simulink model "ImuCalibrator3Pass"  (R2018a)
settings: Solver=FixedStepDiscrete  StartTime=0.0  StopTime=inf  FixedStep=1/Fss  RelTol=1e-3
PreLoadFcn:
  | busDef
  | Fss = 1125;
  | Fss = 2100;
InitFcn:
  | modelDef = getModelDef(true);
undefined symbols (not defined in the file or in its folder): df, dw, Ggyr, Macc, Mgyr, numStates
libraries: simulink x15, vrlib x15, dspsigops x6, dspindex x6, dspinverses x6, dspstat3 x3, simulink_extras x3, dspmtrx3 x3, dspsrcs4 x3, dspmathops x3, dspswit3 x1
(part 2 of 4)

== system ImuCalibrator3Pass/firstPass/AINS/gravity meas update ==
  note: this is just to enforce block execution order
  In1 : Inport
  f_ib^b : Inport  Port=2
  stilltime : Inport  Port=3
  Constant : Constant  Value=eye(3)
  Data Store Read1 : DataStoreRead  DataStoreName=Cbn
  Data Store Read3 : DataStoreRead  DataStoreName=P
  Data Store Write : DataStoreWrite  DataStoreName=P
  MATLAB Function1 : MATLAB Function  TreatAsAtomicUnit=on
  MATLAB Function2 : MATLAB Function  TreatAsAtomicUnit=on
  MATLAB Function3 : MATLAB Function  TreatAsAtomicUnit=on
  Math Function : Math  Operator=reciprocal  SaturateOnIntegerOverflow=on
  Math Function1 : Math  Operator=square  SaturateOnIntegerOverflow=on
  Pad : dspsigops/Pad  padAlong=Rows  dimsToPad=1  valSrc=Specify via dialog  padVal=0  spec=Output size  padNumOutRowsSpecMethod=User-specified  numOutRows=1  padNumOutColsSpecMethod=User-specified  numOutCols=numStates  isVarDimsMode=off  padBeginning=0  padEnd=0  outSizeMode=User-specified  outSize=1  padSigAt=End  trunc_flag=None  roundingMode=Floor  overflowMode=off  truncOrWrapMode=Truncate  wrap_flag=None
      settings: SourceProductName=DSP System Toolbox  SourceProductBaseCode=DS
  Permute Dimensions : PermuteDimensions
  Product : Product  Multiplication=Matrix(*)
  Product1 : Product  Multiplication=Matrix(*)
  Product2 : Product
  Product3 : Product  Multiplication=Matrix(*)
  Saturation : Saturate  UpperLimit=9.8*4  LowerLimit=1
  Sum1 : Sum  Inputs=|+-
  "specific force at rest is up, which is -z in NED frame" : Constant  Value=[ 0; 0; -9.8]
  update the Cbn and b_g with the errors : Subsystem
  Out1 : Outport
  wires:
  In1/1 -> Out1/1
  f_ib^b/1 -> Sum1/1  "when still,  z = Cnb*[0 0 -9.8]' + v"
  Data Store Read1/1 -> Permute Dimensions/1  "Cbn hat"
  Permute Dimensions/1 -> Product3/1, Product/1  "Cnb hat"
  Product/1 -> Sum1/2  "zhat"
  Sum1/1 -> Product1/2  "nu = z-zhat"
  MATLAB Function3/1(Pplus) -> Data Store Write/1
  Product3/1 -> Pad/1
  "specific force at rest is up, which is -z in NED frame"/1 -> MATLAB Function2/1(inp_vr), Product/2
  MATLAB Function2/1(res) -> Product3/2
  Data Store Read3/1 -> MATLAB Function3/1(P), MATLAB Function1/1(P)
  Product2/1 -> MATLAB Function3/4(R), MATLAB Function1/3(R)
  Product1/1 -> update the Cbn and b_g with the errors/1(" error state estimates")  "errors"
  Constant/1 -> Product2/1
  Math Function/1 -> Saturation/1
  Saturation/1 -> Math Function1/1
  stilltime/1 -> Math Function/1
  Math Function1/1 -> Product2/2
  Pad/1 -> MATLAB Function3/3(H), MATLAB Function1/2(H)
  MATLAB Function1/2(K) -> Product1/1, MATLAB Function3/2(K)

== system ImuCalibrator3Pass/firstPass/AINS/initialize states and covariances ==
  stilltime : Inport
  f^b : Inport  Port=2
  Compare To Constant : simulink/Logic and Bit Operations/Compare To Constant  relop=>  const=1.0  OutDataTypeStr=boolean
  Data Store Memory : DataStoreMemory  DataStoreName=INITIALIZED  ReadBeforeWriteMsg=warning  WriteAfterWriteMsg=warning  WriteAfterReadMsg=warning  ShowAdditionalParam=off
  Data Store Read : DataStoreRead  DataStoreName=INITIALIZED
  INITIALIZED = 1 : Subsystem
  Logical Operator : Logic  AllPortsSameDT=off  OutDataTypeStr=boolean
  Logical Operator1 : Logic  Operator=NOT  Inputs=1  IconShape=distinctive  AllPortsSameDT=off  OutDataTypeStr=boolean
  calc Cbn : Subsystem  TreatAsAtomicUnit=on
  set P : Subsystem
  set states : Subsystem  TreatAsAtomicUnit=on
  initializing : Outport
  wires:
  Compare To Constant/1 -> Logical Operator/2
  stilltime/1 -> Compare To Constant/1
  Data Store Read/1 -> Logical Operator1/1
  Logical Operator1/1 -> Logical Operator/1
  f^b/1 -> calc Cbn/1(f^b)
  calc Cbn/2(Cbn) -> set states/1(Cbn)
  INITIALIZED = 1/1(Out1) -> initializing/1
  Logical Operator/1 -> calc Cbn/Enable
  calc Cbn/1(Out1) -> set states/Enable
  set states/1(Out1) -> set P/Enable
  set P/1(Out1) -> INITIALIZED = 1/Enable

== system ImuCalibrator3Pass/firstPass/AINS/report output ==
  In1 : Inport
  w_comp : Inport  Port=2
  f_comp : Inport  Port=3
  Dt : Inport  Port=4
  stilltime : Inport  Port=5
  Bus Creator : BusCreator  Inputs=14
  Data Store Read : DataStoreRead  DataStoreName=Cbn
  Data Store Read1 : DataStoreRead  DataStoreName=P
  Data Store Read2 : DataStoreRead  DataStoreName=dw
  Data Store Read3 : DataStoreRead  DataStoreName=rnav
  Data Store Read4 : DataStoreRead  DataStoreName=vnav
  Data Store Read5 : DataStoreRead  DataStoreName=df
  Data Store Read6 : DataStoreRead  DataStoreName=Mgyr
  Data Store Read7 : DataStoreRead  DataStoreName=Macc
  Data Store Read8 : DataStoreRead  DataStoreName=Ggyr
  Extract Diagonal : dspmtrx3/Extract Diagonal
      settings: SourceProductName=DSP System Toolbox  SourceProductBaseCode=DS
  MATLAB Function1 : MATLAB Function  TreatAsAtomicUnit=on
  MATLAB Function3 : MATLAB Function  TreatAsAtomicUnit=on
  Reshape : Reshape  OutputDimensionality=Column vector (2-D)
  Sqrt : Sqrt  SaturateOnIntegerOverflow=on
  Terminator : Terminator
  filterOut : Outport
  wires:
  Data Store Read/1 -> MATLAB Function1/1(Cbn), MATLAB Function3/1(Cbn)
  Extract Diagonal/1 -> Sqrt/1
  Data Store Read1/1 -> Extract Diagonal/1
  In1/1 -> Terminator/1
  Bus Creator/1 -> filterOut/1
  Data Store Read6/1 -> Bus Creator/10  "Mgyr"
  Sqrt/1 -> Reshape/1  "sigmas"
  f_comp/1 -> Bus Creator/9  "f_comp"
  Data Store Read8/1 -> Bus Creator/12  "Ggyr"
  Data Store Read5/1 -> Bus Creator/6  "df"
  w_comp/1 -> Bus Creator/8  "w_comp"
  Data Store Read4/1 -> Bus Creator/5  "vnav"
  Data Store Read2/1 -> Bus Creator/3  "dw"
  Data Store Read3/1 -> Bus Creator/4  "rnav"
  MATLAB Function3/1(eul) -> Bus Creator/2  "eulers"
  Data Store Read7/1 -> Bus Creator/11  "Macc"
  MATLAB Function1/1(quat) -> Bus Creator/1  "quaternion"
  Dt/1 -> Bus Creator/13  "Dt"
  stilltime/1 -> Bus Creator/14  "stilltime"
  Reshape/1 -> Bus Creator/7  "sigmas"

== system ImuCalibrator3Pass/firstPass/AINS/sensor compensation ==
  note: w_meas = w_true + dw + Mgyr * w_true + Ggyr * f_true
      | w_comp = (I + Mgyr) -1 * (w_meas - dw - Ggyr * f_true)
      |
      | f_meas = f_true + df + Macc * f_true
      | f_comp = (I + Macc) -1 * (f_meas - df)
  w_ib^b : Inport  Unit=rad/s
  f_ib^b : Inport  Port=2  Unit=m/s^2  PortDimensions=3
  Dt : Inport  Port=3  Unit=rad/s
  Data Store Read : DataStoreRead  DataStoreName=IplusMinv_gyr
  Data Store Read1 : DataStoreRead  DataStoreName=dw
  Data Store Read2 : DataStoreRead  DataStoreName=IplusMinv_acc
  Data Store Read3 : DataStoreRead  DataStoreName=df
  Data Store Read4 : DataStoreRead  DataStoreName=Ggyr
  Product : Product  Multiplication=Matrix(*)
  Product1 : Product  Multiplication=Matrix(*)
  Product2 : Product  Multiplication=Matrix(*)
  Sum : Sum  Inputs=|+-
  Sum1 : Sum  Inputs=|+-
  Sum2 : Sum  Inputs=|+-
  w_comp : Outport
  f_comp : Outport  Port=2
  DtOut : Outport  Port=3
  wires:
  Dt/1 -> DtOut/1
  Data Store Read1/1 -> Sum/2
  w_ib^b/1 -> Sum/1
  Sum/1 -> Sum2/1
  Data Store Read/1 -> Product/1
  Product/1 -> w_comp/1
  Product1/1 -> Product2/2, f_comp/1
  Data Store Read2/1 -> Product1/1
  Sum1/1 -> Product1/2
  f_ib^b/1 -> Sum1/1
  Data Store Read3/1 -> Sum1/2
  Sum2/1 -> Product/2
  Product2/1 -> Sum2/2
  Data Store Read4/1 -> Product2/1

== system ImuCalibrator3Pass/firstPass/AINS/time update ==
  Cbn : Inport
  Dt : Inport  Port=2
  w : Inport  Port=3
  f : Inport  Port=4
  Constant : Constant  Commented=on  Value=numStates
  Data Store Read : DataStoreRead  DataStoreName=P
  Data Store Read1 : DataStoreRead  DataStoreName=Cbn
  Data Store Write : DataStoreWrite  DataStoreName=P
  MATLAB Function : MATLAB Function  TreatAsAtomicUnit=on
  MATLAB Function1 : MATLAB Function  Commented=on  TreatAsAtomicUnit=on
  MATLAB Function2 : MATLAB Function  Commented=on  TreatAsAtomicUnit=on
  MATLAB Function3 : MATLAB Function  TreatAsAtomicUnit=on
  Permute Dimensions : PermuteDimensions
  Product2 : Product  Inputs=3  Multiplication=Matrix(*)
  Sum : Sum  Inputs=|++
  Out1 : Outport
  wires:
  Cbn/1 -> Out1/1  "this is just to enforce block execution order"
  Dt/1 -> MATLAB Function3/3(Dt), MATLAB Function/3(Dt)
  MATLAB Function3/1(Phi) -> Permute Dimensions/1, Product2/1  "Phi"
  Data Store Read/1 -> Product2/2
  Permute Dimensions/1 -> Product2/3  "Phi'"
  Sum/1 -> Data Store Write/1  "Phi*P*Phi' + Q"
  Data Store Read1/1 -> MATLAB Function3/4(Cbn), MATLAB Function/4(Cbn)
  w/1 -> MATLAB Function3/1(omega), MATLAB Function/1(omega)
  f/1 -> MATLAB Function3/2(fbod), MATLAB Function/2(f_ib)
  Constant/1 -> MATLAB Function2/1(numStates)
  MATLAB Function/1(Q) -> Sum/2
  Product2/1 -> Sum/1  "Phi*P*Phi'"

== system ImuCalibrator3Pass/firstPass/AINS/zero velocity update ==
  note: this is just to enforce block execution order
  In1 : Inport
  stilltime : Inport  Port=2
  0.01s to 10s : Saturate  UpperLimit=10  LowerLimit=0.01
  Constant : Constant  Value=eye(3)
  Constant1 : Constant  Value=eye(3)
  Constant2 : Constant  Value=zeros(3,9)  VectorParams1D=off
  Constant3 : Constant  Value=zeros(3,1)  VectorParams1D=off
  Data Store Read1 : DataStoreRead  DataStoreName=vnav
  Data Store Read3 : DataStoreRead  DataStoreName=P
  Data Store Write : DataStoreWrite  DataStoreName=P
  MATLAB Function1 : MATLAB Function  TreatAsAtomicUnit=on
  MATLAB Function3 : MATLAB Function  TreatAsAtomicUnit=on
  Math Function : Math  Operator=reciprocal  SaturateOnIntegerOverflow=on
  Math Function1 : Math  Operator=square  SaturateOnIntegerOverflow=on
  Matrix Concatenate : Concatenate  Mode=Multidimensional array  ConcatenateDimension=2
  Pad : dspsigops/Pad  padAlong=Rows  dimsToPad=1  valSrc=Specify via dialog  padVal=0  spec=Output size  padNumOutRowsSpecMethod=User-specified  numOutRows=1  padNumOutColsSpecMethod=User-specified  numOutCols=modelDef.numStates  isVarDimsMode=off  padBeginning=0  padEnd=0  outSizeMode=User-specified  outSize=1  padSigAt=End  trunc_flag=None  roundingMode=Floor  overflowMode=off  truncOrWrapMode=Truncate  wrap_flag=None
      settings: SourceProductName=DSP System Toolbox  SourceProductBaseCode=DS
  Product1 : Product  Multiplication=Matrix(*)
  Product2 : Product
  Saturation : Saturate  UpperLimit=100  LowerLimit=0.1
  Scope : Scope
  Scope1 : Scope
  Sum1 : Sum  Inputs=|+-
  update the underlying states : Subsystem
  Out1 : Outport
  wires:
  MATLAB Function1/2(K) -> Product1/1, MATLAB Function3/2(K)
  Pad/1 -> MATLAB Function1/2(H), MATLAB Function3/3(H)
  Math Function1/1 -> Product2/2
  stilltime/1 -> 0.01s to 10s/1
  Saturation/1 -> Scope/1, Math Function1/1
  Math Function/1 -> Saturation/1
  Constant/1 -> Product2/1
  Product1/1 -> update the underlying states/1(" error state estimates")  "errors"
  Product2/1 -> MATLAB Function1/3(R), MATLAB Function3/4(R)
  Data Store Read3/1 -> MATLAB Function1/1(P), MATLAB Function3/1(P)
  Matrix Concatenate/1 -> Pad/1
  MATLAB Function3/1(Pplus) -> Data Store Write/1
  Sum1/1 -> Scope1/1, Product1/2  "nu = dv = vhat - vtrue"
  In1/1 -> Out1/1
  Constant2/1 -> Matrix Concatenate/1
  Constant1/1 -> Matrix Concatenate/2
  0.01s to 10s/1 -> Math Function/1
  Data Store Read1/1 -> Sum1/1
  Constant3/1 -> Sum1/2

== system ImuCalibrator3Pass/firstPass/readImuData/write SensorTypeIdentifier once ==
  In1 : Inport
  Enable : EnablePort
  Data Store Write : DataStoreWrite  DataStoreName=SensorTypeIdentifier
  wires:
  In1/1 -> Data Store Write/1

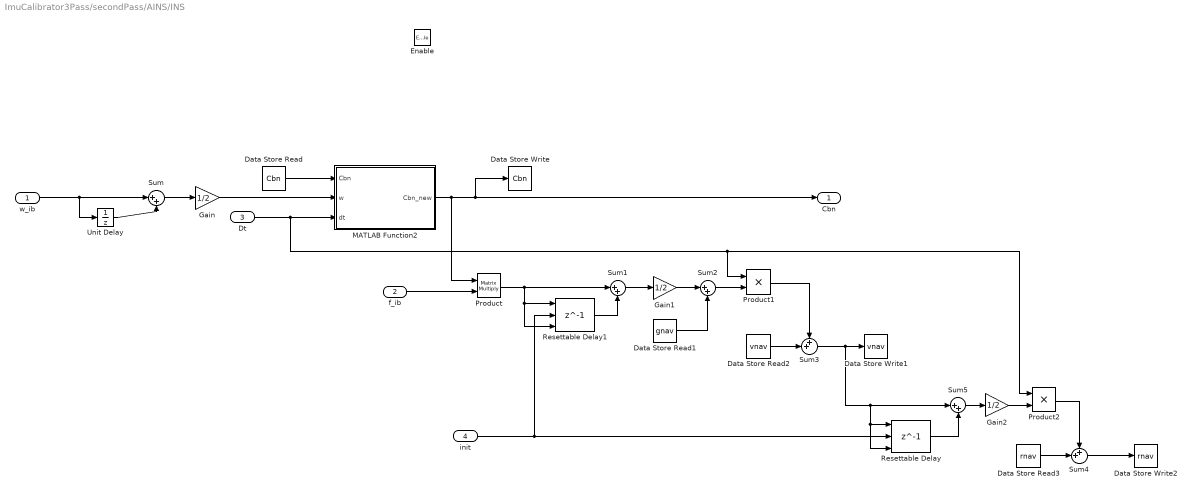
== system ImuCalibrator3Pass/secondPass/AINS/INS ==
  w_ib : Inport
  f_ib : Inport  Port=2
  Dt : Inport  Port=3
  init : Inport  Port=4
  Enable : EnablePort
  Data Store Read : DataStoreRead  DataStoreName=Cbn
  Data Store Read1 : DataStoreRead  DataStoreName=gnav
  Data Store Read2 : DataStoreRead  DataStoreName=vnav
  Data Store Read3 : DataStoreRead  DataStoreName=rnav
  Data Store Write : DataStoreWrite  DataStoreName=Cbn
  Data Store Write1 : DataStoreWrite  DataStoreName=vnav
  Data Store Write2 : DataStoreWrite  DataStoreName=rnav
  Gain : Gain  Gain=1/2
  Gain1 : Gain  Gain=1/2
  Gain2 : Gain  Gain=1/2
  MATLAB Function2 : MATLAB Function  TreatAsAtomicUnit=on
  Product : Product  Multiplication=Matrix(*)
  Product1 : Product
  Product2 : Product
  Resettable Delay : Delay  DelayLength=1  InitialConditionSource=Input port  ExternalReset=Level
      settings: InputPortMap=u0,r5,p4
  Resettable Delay1 : Delay  DelayLength=1  InitialConditionSource=Input port  ExternalReset=Level
      settings: InputPortMap=u0,r5,p4
  Sum{,1..2,5} (4 alike) : Sum  Inputs=|++
  Sum3 : Sum  Inputs=++|
  Sum4 : Sum  Inputs=++|
  Unit Delay : UnitDelay  SampleTime=-1
  Cbn : Outport
  wires:
  Product2/1 -> Sum4/1
  Resettable Delay1/1 -> Sum1/2
  init/1 -> Resettable Delay/2, Resettable Delay1/2
  Resettable Delay/1 -> Sum5/2
  Gain2/1 -> Product2/2
  Sum3/1 -> Data Store Write1/1, Sum5/1, Resettable Delay/1, Resettable Delay/3
  Sum5/1 -> Gain2/1
  Sum4/1 -> Data Store Write2/1
  Data Store Read3/1 -> Sum4/2
  Product1/1 -> Sum3/1
  Data Store Read2/1 -> Sum3/2
  Gain1/1 -> Sum2/1
  Sum1/1 -> Gain1/1
  Product/1 -> Sum1/1, Resettable Delay1/1, Resettable Delay1/3
  Sum2/1 -> Product1/2
  Data Store Read1/1 -> Sum2/2
  f_ib/1 -> Product/2
  Gain/1 -> MATLAB Function2/2(w)
  Sum/1 -> Gain/1
  Unit Delay/1 -> Sum/2
  MATLAB Function2/1(Cbn_new) -> Data Store Write/1, Cbn/1, Product/1
  w_ib/1 -> Sum/1, Unit Delay/1
  Data Store Read/1 -> MATLAB Function2/1(Cbn)
  Dt/1 -> MATLAB Function2/3(dt), Product1/1, Product2/1

== system ImuCalibrator3Pass/secondPass/AINS/compass meas update ==
  note: this is just to enforce block execution order
  In1 : Inport
  m^b : Inport  Port=2
  Enable : EnablePort
  Data Store Read1 : DataStoreRead  DataStoreName=Cbn
  Data Store Read3 : DataStoreRead  DataStoreName=P
  Data Store Write : DataStoreWrite  DataStoreName=P
  Demux : Demux  Outputs=3
  Gain : Gain  Gain=-1
  H : Constant  Value=[ 0 0 1]  VectorParams1D=off
  MATLAB Function1 : MATLAB Function  TreatAsAtomicUnit=on
  MATLAB Function3 : MATLAB Function  TreatAsAtomicUnit=on
  Product : Product  Multiplication=Matrix(*)
  Product1 : Product  Multiplication=Matrix(*)
  R assumes 10 deg rms compass noise : Constant  Value=0.34^2
  Scope : Scope
  Scope1 : Scope
  Scope2 : Scope
  Trigonometric Function : Trigonometry  Operator=atan2
  update the Cbn with the errors : Subsystem
  Out1 : Outport
  wires:
  Gain/1 -> Scope1/1, Product1/2
  H/1 -> MATLAB Function3/3(H), MATLAB Function1/2(H)
  Demux/1 -> Trigonometric Function/2
  Demux/2 -> Trigonometric Function/1
  In1/1 -> Out1/1
  Data Store Read1/1 -> Product/1  "Cbn hat"
  Product/1 -> Demux/1  "m^nhat"
  Trigonometric Function/1 -> Gain/1  "nu = 0 - psi"
  MATLAB Function1/2(K) -> Scope2/1, MATLAB Function3/2(K), Product1/1
  MATLAB Function3/1(Pplus) -> Data Store Write/1
  m^b/1 -> Product/2
  Data Store Read3/1 -> MATLAB Function3/1(P), MATLAB Function1/1(P)
  R assumes 10 deg rms compass noise/1 -> MATLAB Function3/4(R), MATLAB Function1/3(R)
  Product1/1 -> Scope/1, update the Cbn with the errors/1(phi  rotation errors)  "phi  rotation errors"

== system ImuCalibrator3Pass/secondPass/AINS/gravity meas update ==
  note: this is just to enforce block execution order
  In1 : Inport
  f_ib^b : Inport  Port=2
  stilltime : Inport  Port=3
  Constant : Constant  Value=eye(3)
  Data Store Read1 : DataStoreRead  DataStoreName=Cbn
  Data Store Read3 : DataStoreRead  DataStoreName=P
  Data Store Write : DataStoreWrite  DataStoreName=P
  MATLAB Function1 : MATLAB Function  TreatAsAtomicUnit=on
  MATLAB Function2 : MATLAB Function  TreatAsAtomicUnit=on
  MATLAB Function3 : MATLAB Function  TreatAsAtomicUnit=on
  Math Function : Math  Operator=reciprocal  SaturateOnIntegerOverflow=on
  Math Function1 : Math  Operator=square  SaturateOnIntegerOverflow=on
  Pad : dspsigops/Pad  padAlong=Rows  dimsToPad=1  valSrc=Specify via dialog  padVal=0  spec=Output size  padNumOutRowsSpecMethod=User-specified  numOutRows=1  padNumOutColsSpecMethod=User-specified  numOutCols=numStates  isVarDimsMode=off  padBeginning=0  padEnd=0  outSizeMode=User-specified  outSize=1  padSigAt=End  trunc_flag=None  roundingMode=Floor  overflowMode=off  truncOrWrapMode=Truncate  wrap_flag=None
      settings: SourceProductName=DSP System Toolbox  SourceProductBaseCode=DS
  Permute Dimensions : PermuteDimensions
  Product : Product  Multiplication=Matrix(*)
  Product1 : Product  Multiplication=Matrix(*)
  Product2 : Product
  Product3 : Product  Multiplication=Matrix(*)
  Saturation : Saturate  UpperLimit=9.8*4  LowerLimit=1
  Sum1 : Sum  Inputs=|+-
  "specific force at rest is up, which is -z in NED frame" : Constant  Value=[ 0; 0; -9.8]
  update the Cbn and b_g with the errors : Subsystem
  Out1 : Outport
  wires:
  MATLAB Function1/2(K) -> MATLAB Function3/2(K), Product1/1
  Pad/1 -> MATLAB Function1/2(H), MATLAB Function3/3(H)
  Math Function1/1 -> Product2/2
  stilltime/1 -> Math Function/1
  Saturation/1 -> Math Function1/1
  Math Function/1 -> Saturation/1
  Constant/1 -> Product2/1
  Product1/1 -> update the Cbn and b_g with the errors/1(" error state estimates")  "errors"
  Product2/1 -> MATLAB Function1/3(R), MATLAB Function3/4(R)
  Data Store Read3/1 -> MATLAB Function1/1(P), MATLAB Function3/1(P)
  MATLAB Function2/1(res) -> Product3/2
  "specific force at rest is up, which is -z in NED frame"/1 -> Product/2, MATLAB Function2/1(inp_vr)
  Product3/1 -> Pad/1
  MATLAB Function3/1(Pplus) -> Data Store Write/1
  Sum1/1 -> Product1/2  "nu = z-zhat"
  Product/1 -> Sum1/2  "zhat"
  Permute Dimensions/1 -> Product/1, Product3/1  "Cnb hat"
  Data Store Read1/1 -> Permute Dimensions/1  "Cbn hat"
  f_ib^b/1 -> Sum1/1  "when still,  z = Cnb*[0 0 -9.8]' + v"
  In1/1 -> Out1/1

== system ImuCalibrator3Pass/secondPass/AINS/initialize states and covariances ==
  stilltime : Inport
  f^b : Inport  Port=2
  Compare To Constant : simulink/Logic and Bit Operations/Compare To Constant  relop=>  const=1.0  OutDataTypeStr=boolean
  Data Store Memory : DataStoreMemory  DataStoreName=INITIALIZED  ReadBeforeWriteMsg=warning  WriteAfterWriteMsg=warning  WriteAfterReadMsg=warning  ShowAdditionalParam=off
  Data Store Read : DataStoreRead  DataStoreName=INITIALIZED
  INITIALIZED = 1 : Subsystem
  Logical Operator : Logic  AllPortsSameDT=off  OutDataTypeStr=boolean
  Logical Operator1 : Logic  Operator=NOT  Inputs=1  IconShape=distinctive  AllPortsSameDT=off  OutDataTypeStr=boolean
  calc Cbn : Subsystem  TreatAsAtomicUnit=on
  set P : Subsystem
  set states : Subsystem  TreatAsAtomicUnit=on
  initializing : Outport
  wires:
  set P/1(Out1) -> INITIALIZED = 1/Enable
  set states/1(Out1) -> set P/Enable
  calc Cbn/1(Out1) -> set states/Enable
  Logical Operator/1 -> calc Cbn/Enable
  INITIALIZED = 1/1(Out1) -> initializing/1
  calc Cbn/2(Cbn) -> set states/1(Cbn)
  f^b/1 -> calc Cbn/1(f^b)
  Logical Operator1/1 -> Logical Operator/1
  Data Store Read/1 -> Logical Operator1/1
  stilltime/1 -> Compare To Constant/1
  Compare To Constant/1 -> Logical Operator/2

== system ImuCalibrator3Pass/secondPass/AINS/report output ==
  In1 : Inport
  w_comp : Inport  Port=2
  f_comp : Inport  Port=3
  Dt : Inport  Port=4
  stilltime : Inport  Port=5
  Bus Creator : BusCreator  Inputs=14
  Data Store Read : DataStoreRead  DataStoreName=Cbn
  Data Store Read1 : DataStoreRead  DataStoreName=P
  Data Store Read2 : DataStoreRead  DataStoreName=dw
  Data Store Read3 : DataStoreRead  DataStoreName=rnav
  Data Store Read4 : DataStoreRead  DataStoreName=vnav
  Data Store Read5 : DataStoreRead  DataStoreName=df
  Data Store Read6 : DataStoreRead  DataStoreName=Mgyr
  Data Store Read7 : DataStoreRead  DataStoreName=Macc
  Data Store Read8 : DataStoreRead  DataStoreName=Ggyr
  Extract Diagonal : dspmtrx3/Extract Diagonal
      settings: SourceProductName=DSP System Toolbox  SourceProductBaseCode=DS
  MATLAB Function1 : MATLAB Function  TreatAsAtomicUnit=on
  MATLAB Function3 : MATLAB Function  TreatAsAtomicUnit=on
  Reshape : Reshape  OutputDimensionality=Column vector (2-D)
  Sqrt : Sqrt  SaturateOnIntegerOverflow=on
  Terminator : Terminator
  filterOut : Outport
  wires:
  Reshape/1 -> Bus Creator/7  "sigmas"
  stilltime/1 -> Bus Creator/14  "stilltime"
  Dt/1 -> Bus Creator/13  "Dt"
  MATLAB Function1/1(quat) -> Bus Creator/1  "quaternion"
  Data Store Read7/1 -> Bus Creator/11  "Macc"
  MATLAB Function3/1(eul) -> Bus Creator/2  "eulers"
  Data Store Read3/1 -> Bus Creator/4  "rnav"
  Data Store Read2/1 -> Bus Creator/3  "dw"
  Data Store Read4/1 -> Bus Creator/5  "vnav"
  w_comp/1 -> Bus Creator/8  "w_comp"
  Data Store Read5/1 -> Bus Creator/6  "df"
  Data Store Read8/1 -> Bus Creator/12  "Ggyr"
  f_comp/1 -> Bus Creator/9  "f_comp"
  Sqrt/1 -> Reshape/1  "sigmas"
  Data Store Read6/1 -> Bus Creator/10  "Mgyr"
  Bus Creator/1 -> filterOut/1
  In1/1 -> Terminator/1
  Data Store Read1/1 -> Extract Diagonal/1
  Extract Diagonal/1 -> Sqrt/1
  Data Store Read/1 -> MATLAB Function3/1(Cbn), MATLAB Function1/1(Cbn)

== system ImuCalibrator3Pass/secondPass/AINS/sensor compensation ==
  note: w_meas = w_true + dw + Mgyr * w_true + Ggyr * f_true
      | w_comp = (I + Mgyr) -1 * (w_meas - dw - Ggyr * f_true)
      |
      | f_meas = f_true + df + Macc * f_true
      | f_comp = (I + Macc) -1 * (f_meas - df)
  w_ib^b : Inport  Unit=rad/s
  f_ib^b : Inport  Port=2  Unit=m/s^2  PortDimensions=3
  Dt : Inport  Port=3  Unit=rad/s
  Data Store Read : DataStoreRead  DataStoreName=IplusMinv_gyr
  Data Store Read1 : DataStoreRead  DataStoreName=dw
  Data Store Read2 : DataStoreRead  DataStoreName=IplusMinv_acc
  Data Store Read3 : DataStoreRead  DataStoreName=df
  Data Store Read4 : DataStoreRead  DataStoreName=Ggyr
  Product : Product  Multiplication=Matrix(*)
  Product1 : Product  Multiplication=Matrix(*)
  Product2 : Product  Multiplication=Matrix(*)
  Sum : Sum  Inputs=|+-
  Sum1 : Sum  Inputs=|+-
  Sum2 : Sum  Inputs=|+-
  w_comp : Outport
  f_comp : Outport  Port=2
  DtOut : Outport  Port=3
  wires:
  Data Store Read4/1 -> Product2/1
  Product2/1 -> Sum2/2
  Sum2/1 -> Product/2
  Data Store Read3/1 -> Sum1/2
  f_ib^b/1 -> Sum1/1
  Sum1/1 -> Product1/2
  Data Store Read2/1 -> Product1/1
  Product1/1 -> f_comp/1, Product2/2
  Product/1 -> w_comp/1
  Data Store Read/1 -> Product/1
  Sum/1 -> Sum2/1
  w_ib^b/1 -> Sum/1
  Data Store Read1/1 -> Sum/2
  Dt/1 -> DtOut/1

== system ImuCalibrator3Pass/secondPass/AINS/time update ==
  Cbn : Inport
  Dt : Inport  Port=2
  w : Inport  Port=3
  f : Inport  Port=4
  Constant : Constant  Commented=on  Value=numStates
  Data Store Read : DataStoreRead  DataStoreName=P
  Data Store Read1 : DataStoreRead  DataStoreName=Cbn
  Data Store Write : DataStoreWrite  DataStoreName=P
  MATLAB Function : MATLAB Function  TreatAsAtomicUnit=on
  MATLAB Function1 : MATLAB Function  Commented=on  TreatAsAtomicUnit=on
  MATLAB Function2 : MATLAB Function  Commented=on  TreatAsAtomicUnit=on
  MATLAB Function3 : MATLAB Function  TreatAsAtomicUnit=on
  Permute Dimensions : PermuteDimensions
  Product2 : Product  Inputs=3  Multiplication=Matrix(*)
  Sum : Sum  Inputs=|++
  Out1 : Outport
  wires:
  Product2/1 -> Sum/1  "Phi*P*Phi'"
  MATLAB Function/1(Q) -> Sum/2
  Constant/1 -> MATLAB Function2/1(numStates)
  f/1 -> MATLAB Function/2(f_ib), MATLAB Function3/2(fbod)
  w/1 -> MATLAB Function/1(omega), MATLAB Function3/1(omega)
  Data Store Read1/1 -> MATLAB Function/4(Cbn), MATLAB Function3/4(Cbn)
  Sum/1 -> Data Store Write/1  "Phi*P*Phi' + Q"
  Permute Dimensions/1 -> Product2/3  "Phi'"
  Data Store Read/1 -> Product2/2
  MATLAB Function3/1(Phi) -> Product2/1, Permute Dimensions/1  "Phi"
  Dt/1 -> MATLAB Function/3(Dt), MATLAB Function3/3(Dt)
  Cbn/1 -> Out1/1  "this is just to enforce block execution order"

== system ImuCalibrator3Pass/secondPass/AINS/zero velocity update ==
  note: this is just to enforce block execution order
  In1 : Inport
  stilltime : Inport  Port=2
  0.01s to 10s : Saturate  UpperLimit=10  LowerLimit=0.01
  Constant : Constant  Value=eye(3)
  Constant1 : Constant  Value=eye(3)
  Constant2 : Constant  Value=zeros(3,9)  VectorParams1D=off
  Constant3 : Constant  Value=zeros(3,1)  VectorParams1D=off
  Data Store Read1 : DataStoreRead  DataStoreName=vnav
  Data Store Read3 : DataStoreRead  DataStoreName=P
  Data Store Write : DataStoreWrite  DataStoreName=P
  MATLAB Function1 : MATLAB Function  TreatAsAtomicUnit=on
  MATLAB Function3 : MATLAB Function  TreatAsAtomicUnit=on
  Math Function : Math  Operator=reciprocal  SaturateOnIntegerOverflow=on
  Math Function1 : Math  Operator=square  SaturateOnIntegerOverflow=on
  Matrix Concatenate : Concatenate  Mode=Multidimensional array  ConcatenateDimension=2
  Pad : dspsigops/Pad  padAlong=Rows  dimsToPad=1  valSrc=Specify via dialog  padVal=0  spec=Output size  padNumOutRowsSpecMethod=User-specified  numOutRows=1  padNumOutColsSpecMethod=User-specified  numOutCols=modelDef.numStates  isVarDimsMode=off  padBeginning=0  padEnd=0  outSizeMode=User-specified  outSize=1  padSigAt=End  trunc_flag=None  roundingMode=Floor  overflowMode=off  truncOrWrapMode=Truncate  wrap_flag=None
      settings: SourceProductName=DSP System Toolbox  SourceProductBaseCode=DS
  Product1 : Product  Multiplication=Matrix(*)
  Product2 : Product
  Saturation : Saturate  UpperLimit=100  LowerLimit=0.1
  Scope : Scope
  Scope1 : Scope
  Sum1 : Sum  Inputs=|+-
  update the underlying states : Subsystem
  Out1 : Outport
  wires:
  Constant3/1 -> Sum1/2
  Data Store Read1/1 -> Sum1/1
  0.01s to 10s/1 -> Math Function/1
  Constant1/1 -> Matrix Concatenate/2
  Constant2/1 -> Matrix Concatenate/1
  In1/1 -> Out1/1
  Sum1/1 -> Product1/2, Scope1/1  "nu = dv = vhat - vtrue"
  MATLAB Function3/1(Pplus) -> Data Store Write/1
  Matrix Concatenate/1 -> Pad/1
  Data Store Read3/1 -> MATLAB Function3/1(P), MATLAB Function1/1(P)
  Product2/1 -> MATLAB Function3/4(R), MATLAB Function1/3(R)
  Product1/1 -> update the underlying states/1(" error state estimates")  "errors"
  Constant/1 -> Product2/1
  Math Function/1 -> Saturation/1
  Saturation/1 -> Math Function1/1, Scope/1
  stilltime/1 -> 0.01s to 10s/1
  Math Function1/1 -> Product2/2
  Pad/1 -> MATLAB Function3/3(H), MATLAB Function1/2(H)
  MATLAB Function1/2(K) -> MATLAB Function3/2(K), Product1/1

== system ImuCalibrator3Pass/secondPass/readImuData/write SensorTypeIdentifier once ==
  In1 : Inport
  Enable : EnablePort
  Data Store Write : DataStoreWrite  DataStoreName=SensorTypeIdentifier
  wires:
  In1/1 -> Data Store Write/1

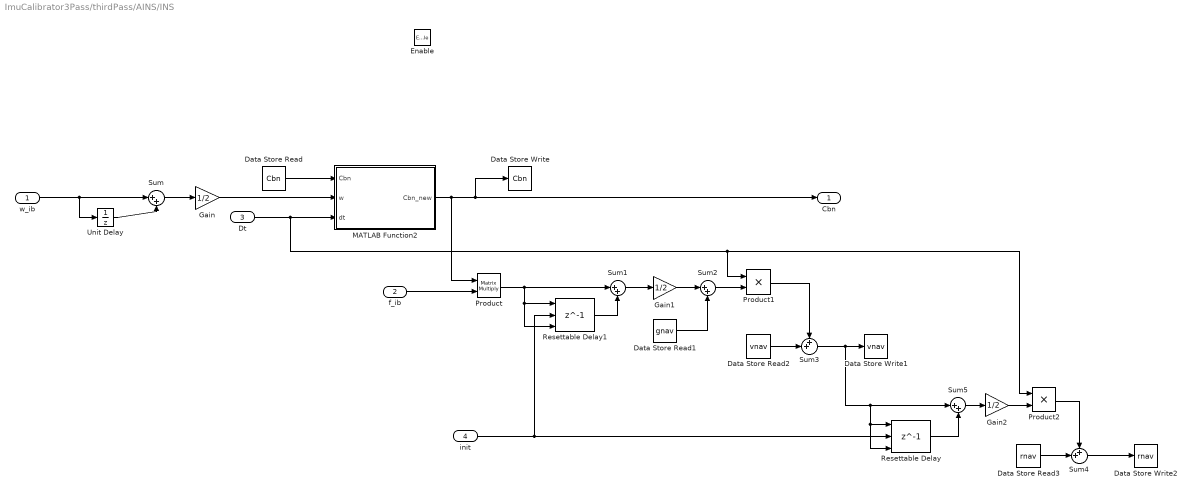
== system ImuCalibrator3Pass/thirdPass/AINS/INS ==
  w_ib : Inport
  f_ib : Inport  Port=2
  Dt : Inport  Port=3
  init : Inport  Port=4
  Enable : EnablePort
  Data Store Read : DataStoreRead  DataStoreName=Cbn
  Data Store Read1 : DataStoreRead  DataStoreName=gnav
  Data Store Read2 : DataStoreRead  DataStoreName=vnav
  Data Store Read3 : DataStoreRead  DataStoreName=rnav
  Data Store Write : DataStoreWrite  DataStoreName=Cbn
  Data Store Write1 : DataStoreWrite  DataStoreName=vnav
  Data Store Write2 : DataStoreWrite  DataStoreName=rnav
  Gain : Gain  Gain=1/2
  Gain1 : Gain  Gain=1/2
  Gain2 : Gain  Gain=1/2
  MATLAB Function2 : MATLAB Function  TreatAsAtomicUnit=on
  Product : Product  Multiplication=Matrix(*)
  Product1 : Product
  Product2 : Product
  Resettable Delay : Delay  DelayLength=1  InitialConditionSource=Input port  ExternalReset=Level
      settings: InputPortMap=u0,r5,p4
  Resettable Delay1 : Delay  DelayLength=1  InitialConditionSource=Input port  ExternalReset=Level
      settings: InputPortMap=u0,r5,p4
  Sum{,1..2,5} (4 alike) : Sum  Inputs=|++
  Sum3 : Sum  Inputs=++|
  Sum4 : Sum  Inputs=++|
  Unit Delay : UnitDelay  SampleTime=-1
  Cbn : Outport
  wires:
  Dt/1 -> Product2/1, Product1/1, MATLAB Function2/3(dt)
  Data Store Read/1 -> MATLAB Function2/1(Cbn)
  w_ib/1 -> Unit Delay/1, Sum/1
  MATLAB Function2/1(Cbn_new) -> Product/1, Cbn/1, Data Store Write/1
  Unit Delay/1 -> Sum/2
  Sum/1 -> Gain/1
  Gain/1 -> MATLAB Function2/2(w)
  f_ib/1 -> Product/2
  Data Store Read1/1 -> Sum2/2
  Sum2/1 -> Product1/2
  Product/1 -> Resettable Delay1/3, Resettable Delay1/1, Sum1/1
  Sum1/1 -> Gain1/1
  Gain1/1 -> Sum2/1
  Data Store Read2/1 -> Sum3/2
  Product1/1 -> Sum3/1
  Data Store Read3/1 -> Sum4/2
  Sum4/1 -> Data Store Write2/1
  Sum5/1 -> Gain2/1
  Sum3/1 -> Resettable Delay/3, Resettable Delay/1, Sum5/1, Data Store Write1/1
  Gain2/1 -> Product2/2
  Resettable Delay/1 -> Sum5/2
  init/1 -> Resettable Delay1/2, Resettable Delay/2
  Resettable Delay1/1 -> Sum1/2
  Product2/1 -> Sum4/1

== system ImuCalibrator3Pass/thirdPass/AINS/compass meas update ==
  note: this is just to enforce block execution order
  In1 : Inport
  m^b : Inport  Port=2
  Enable : EnablePort
  Data Store Read1 : DataStoreRead  DataStoreName=Cbn
  Data Store Read3 : DataStoreRead  DataStoreName=P
  Data Store Write : DataStoreWrite  DataStoreName=P
  Demux : Demux  Outputs=3
  Gain : Gain  Gain=-1
  H : Constant  Value=[ 0 0 1]  VectorParams1D=off
  MATLAB Function1 : MATLAB Function  TreatAsAtomicUnit=on
  MATLAB Function3 : MATLAB Function  TreatAsAtomicUnit=on
  Product : Product  Multiplication=Matrix(*)
  Product1 : Product  Multiplication=Matrix(*)
  R assumes 10 deg rms compass noise : Constant  Value=0.34^2
  Scope : Scope
  Scope1 : Scope
  Scope2 : Scope
  Trigonometric Function : Trigonometry  Operator=atan2
  update the Cbn with the errors : Subsystem
  Out1 : Outport
  wires:
  Product1/1 -> update the Cbn with the errors/1(phi  rotation errors), Scope/1  "phi  rotation errors"
  R assumes 10 deg rms compass noise/1 -> MATLAB Function1/3(R), MATLAB Function3/4(R)
  Data Store Read3/1 -> MATLAB Function1/1(P), MATLAB Function3/1(P)
  m^b/1 -> Product/2
  MATLAB Function3/1(Pplus) -> Data Store Write/1
  MATLAB Function1/2(K) -> Product1/1, MATLAB Function3/2(K), Scope2/1
  Trigonometric Function/1 -> Gain/1  "nu = 0 - psi"
  Product/1 -> Demux/1  "m^nhat"
  Data Store Read1/1 -> Product/1  "Cbn hat"
  In1/1 -> Out1/1
  Demux/2 -> Trigonometric Function/1
  Demux/1 -> Trigonometric Function/2
  H/1 -> MATLAB Function1/2(H), MATLAB Function3/3(H)
  Gain/1 -> Product1/2, Scope1/1

== system ImuCalibrator3Pass/thirdPass/AINS/gravity meas update ==
  note: this is just to enforce block execution order
  In1 : Inport
  f_ib^b : Inport  Port=2
  stilltime : Inport  Port=3
  Constant : Constant  Value=eye(3)
  Data Store Read1 : DataStoreRead  DataStoreName=Cbn
  Data Store Read3 : DataStoreRead  DataStoreName=P
  Data Store Write : DataStoreWrite  DataStoreName=P
  MATLAB Function1 : MATLAB Function  TreatAsAtomicUnit=on
  MATLAB Function2 : MATLAB Function  TreatAsAtomicUnit=on
  MATLAB Function3 : MATLAB Function  TreatAsAtomicUnit=on
  Math Function : Math  Operator=reciprocal  SaturateOnIntegerOverflow=on
  Math Function1 : Math  Operator=square  SaturateOnIntegerOverflow=on
  Pad : dspsigops/Pad  padAlong=Rows  dimsToPad=1  valSrc=Specify via dialog  padVal=0  spec=Output size  padNumOutRowsSpecMethod=User-specified  numOutRows=1  padNumOutColsSpecMethod=User-specified  numOutCols=numStates  isVarDimsMode=off  padBeginning=0  padEnd=0  outSizeMode=User-specified  outSize=1  padSigAt=End  trunc_flag=None  roundingMode=Floor  overflowMode=off  truncOrWrapMode=Truncate  wrap_flag=None
      settings: SourceProductName=DSP System Toolbox  SourceProductBaseCode=DS
  Permute Dimensions : PermuteDimensions
  Product : Product  Multiplication=Matrix(*)
  Product1 : Product  Multiplication=Matrix(*)
  Product2 : Product
  Product3 : Product  Multiplication=Matrix(*)
  Saturation : Saturate  UpperLimit=9.8*4  LowerLimit=1
  Sum1 : Sum  Inputs=|+-
  "specific force at rest is up, which is -z in NED frame" : Constant  Value=[ 0; 0; -9.8]
  update the Cbn and b_g with the errors : Subsystem
  Out1 : Outport
  wires:
  In1/1 -> Out1/1
  f_ib^b/1 -> Sum1/1  "when still,  z = Cnb*[0 0 -9.8]' + v"
  Data Store Read1/1 -> Permute Dimensions/1  "Cbn hat"
  Permute Dimensions/1 -> Product3/1, Product/1  "Cnb hat"
  Product/1 -> Sum1/2  "zhat"
  Sum1/1 -> Product1/2  "nu = z-zhat"
  MATLAB Function3/1(Pplus) -> Data Store Write/1
  Product3/1 -> Pad/1
  "specific force at rest is up, which is -z in NED frame"/1 -> MATLAB Function2/1(inp_vr), Product/2
  MATLAB Function2/1(res) -> Product3/2
  Data Store Read3/1 -> MATLAB Function3/1(P), MATLAB Function1/1(P)
  Product2/1 -> MATLAB Function3/4(R), MATLAB Function1/3(R)
  Product1/1 -> update the Cbn and b_g with the errors/1(" error state estimates")  "errors"
  Constant/1 -> Product2/1
  Math Function/1 -> Saturation/1
  Saturation/1 -> Math Function1/1
  stilltime/1 -> Math Function/1
  Math Function1/1 -> Product2/2
  Pad/1 -> MATLAB Function3/3(H), MATLAB Function1/2(H)
  MATLAB Function1/2(K) -> Product1/1, MATLAB Function3/2(K)

== system ImuCalibrator3Pass/thirdPass/AINS/initialize states and covariances ==
  stilltime : Inport
  f^b : Inport  Port=2
  Compare To Constant : simulink/Logic and Bit Operations/Compare To Constant  relop=>  const=1.0  OutDataTypeStr=boolean
  Data Store Memory : DataStoreMemory  DataStoreName=INITIALIZED  ReadBeforeWriteMsg=warning  WriteAfterWriteMsg=warning  WriteAfterReadMsg=warning  ShowAdditionalParam=off
  Data Store Read : DataStoreRead  DataStoreName=INITIALIZED
  INITIALIZED = 1 : Subsystem
  Logical Operator : Logic  AllPortsSameDT=off  OutDataTypeStr=boolean
  Logical Operator1 : Logic  Operator=NOT  Inputs=1  IconShape=distinctive  AllPortsSameDT=off  OutDataTypeStr=boolean
  calc Cbn : Subsystem  TreatAsAtomicUnit=on
  set P : Subsystem
  set states : Subsystem  TreatAsAtomicUnit=on
  initializing : Outport
  wires:
  Compare To Constant/1 -> Logical Operator/2
  stilltime/1 -> Compare To Constant/1
  Data Store Read/1 -> Logical Operator1/1
  Logical Operator1/1 -> Logical Operator/1
  f^b/1 -> calc Cbn/1(f^b)
  calc Cbn/2(Cbn) -> set states/1(Cbn)
  INITIALIZED = 1/1(Out1) -> initializing/1
  Logical Operator/1 -> calc Cbn/Enable
  calc Cbn/1(Out1) -> set states/Enable
  set states/1(Out1) -> set P/Enable
  set P/1(Out1) -> INITIALIZED = 1/Enable

== system ImuCalibrator3Pass/thirdPass/AINS/report output ==
  In1 : Inport
  w_comp : Inport  Port=2
  f_comp : Inport  Port=3
  Dt : Inport  Port=4
  stilltime : Inport  Port=5
  Bus Creator : BusCreator  Inputs=14
  Data Store Read : DataStoreRead  DataStoreName=Cbn
  Data Store Read1 : DataStoreRead  DataStoreName=P
  Data Store Read2 : DataStoreRead  DataStoreName=dw
  Data Store Read3 : DataStoreRead  DataStoreName=rnav
  Data Store Read4 : DataStoreRead  DataStoreName=vnav
  Data Store Read5 : DataStoreRead  DataStoreName=df
  Data Store Read6 : DataStoreRead  DataStoreName=Mgyr
  Data Store Read7 : DataStoreRead  DataStoreName=Macc
  Data Store Read8 : DataStoreRead  DataStoreName=Ggyr
  Extract Diagonal : dspmtrx3/Extract Diagonal
      settings: SourceProductName=DSP System Toolbox  SourceProductBaseCode=DS
  MATLAB Function1 : MATLAB Function  TreatAsAtomicUnit=on
  MATLAB Function3 : MATLAB Function  TreatAsAtomicUnit=on
  Reshape : Reshape  OutputDimensionality=Column vector (2-D)
  Sqrt : Sqrt  SaturateOnIntegerOverflow=on
  Terminator : Terminator
  filterOut : Outport
  wires:
  Data Store Read/1 -> MATLAB Function1/1(Cbn), MATLAB Function3/1(Cbn)
  Extract Diagonal/1 -> Sqrt/1
  Data Store Read1/1 -> Extract Diagonal/1
  In1/1 -> Terminator/1
  Bus Creator/1 -> filterOut/1
  Data Store Read6/1 -> Bus Creator/10  "Mgyr"
  Sqrt/1 -> Reshape/1  "sigmas"
  f_comp/1 -> Bus Creator/9  "f_comp"
  Data Store Read8/1 -> Bus Creator/12  "Ggyr"
  Data Store Read5/1 -> Bus Creator/6  "df"
  w_comp/1 -> Bus Creator/8  "w_comp"
  Data Store Read4/1 -> Bus Creator/5  "vnav"
  Data Store Read2/1 -> Bus Creator/3  "dw"
  Data Store Read3/1 -> Bus Creator/4  "rnav"
  MATLAB Function3/1(eul) -> Bus Creator/2  "eulers"
  Data Store Read7/1 -> Bus Creator/11  "Macc"
  MATLAB Function1/1(quat) -> Bus Creator/1  "quaternion"
  Dt/1 -> Bus Creator/13  "Dt"
  stilltime/1 -> Bus Creator/14  "stilltime"
  Reshape/1 -> Bus Creator/7  "sigmas"

== system ImuCalibrator3Pass/thirdPass/AINS/sensor compensation ==
  note: w_meas = w_true + dw + Mgyr * w_true + Ggyr * f_true
      | w_comp = (I + Mgyr) -1 * (w_meas - dw - Ggyr * f_true)
      |
      | f_meas = f_true + df + Macc * f_true
      | f_comp = (I + Macc) -1 * (f_meas - df)
  w_ib^b : Inport  Unit=rad/s
  f_ib^b : Inport  Port=2  Unit=m/s^2  PortDimensions=3
  Dt : Inport  Port=3  Unit=rad/s
  Data Store Read : DataStoreRead  DataStoreName=IplusMinv_gyr
  Data Store Read1 : DataStoreRead  DataStoreName=dw
  Data Store Read2 : DataStoreRead  DataStoreName=IplusMinv_acc
  Data Store Read3 : DataStoreRead  DataStoreName=df
  Data Store Read4 : DataStoreRead  DataStoreName=Ggyr
  Product : Product  Multiplication=Matrix(*)
  Product1 : Product  Multiplication=Matrix(*)
  Product2 : Product  Multiplication=Matrix(*)
  Sum : Sum  Inputs=|+-
  Sum1 : Sum  Inputs=|+-
  Sum2 : Sum  Inputs=|+-
  w_comp : Outport
  f_comp : Outport  Port=2
  DtOut : Outport  Port=3
  wires:
  Dt/1 -> DtOut/1
  Data Store Read1/1 -> Sum/2
  w_ib^b/1 -> Sum/1
  Sum/1 -> Sum2/1
  Data Store Read/1 -> Product/1
  Product/1 -> w_comp/1
  Product1/1 -> Product2/2, f_comp/1
  Data Store Read2/1 -> Product1/1
  Sum1/1 -> Product1/2
  f_ib^b/1 -> Sum1/1
  Data Store Read3/1 -> Sum1/2
  Sum2/1 -> Product/2
  Product2/1 -> Sum2/2
  Data Store Read4/1 -> Product2/1

== system ImuCalibrator3Pass/thirdPass/AINS/time update ==
  Cbn : Inport
  Dt : Inport  Port=2
  w : Inport  Port=3
  f : Inport  Port=4
  Constant : Constant  Commented=on  Value=numStates
  Data Store Read : DataStoreRead  DataStoreName=P
  Data Store Read1 : DataStoreRead  DataStoreName=Cbn
  Data Store Write : DataStoreWrite  DataStoreName=P
  MATLAB Function : MATLAB Function  TreatAsAtomicUnit=on
  MATLAB Function1 : MATLAB Function  Commented=on  TreatAsAtomicUnit=on
  MATLAB Function2 : MATLAB Function  Commented=on  TreatAsAtomicUnit=on
  MATLAB Function3 : MATLAB Function  TreatAsAtomicUnit=on
  Permute Dimensions : PermuteDimensions
  Product2 : Product  Inputs=3  Multiplication=Matrix(*)
  Sum : Sum  Inputs=|++
  Out1 : Outport
  wires:
  Cbn/1 -> Out1/1  "this is just to enforce block execution order"
  Dt/1 -> MATLAB Function3/3(Dt), MATLAB Function/3(Dt)
  MATLAB Function3/1(Phi) -> Permute Dimensions/1, Product2/1  "Phi"
  Data Store Read/1 -> Product2/2
  Permute Dimensions/1 -> Product2/3  "Phi'"
  Sum/1 -> Data Store Write/1  "Phi*P*Phi' + Q"
  Data Store Read1/1 -> MATLAB Function3/4(Cbn), MATLAB Function/4(Cbn)
  w/1 -> MATLAB Function3/1(omega), MATLAB Function/1(omega)
  f/1 -> MATLAB Function3/2(fbod), MATLAB Function/2(f_ib)
  Constant/1 -> MATLAB Function2/1(numStates)
  MATLAB Function/1(Q) -> Sum/2
  Product2/1 -> Sum/1  "Phi*P*Phi'"

== system ImuCalibrator3Pass/thirdPass/AINS/zero velocity update ==
  note: this is just to enforce block execution order
  In1 : Inport
  stilltime : Inport  Port=2
  0.01s to 10s : Saturate  UpperLimit=10  LowerLimit=0.01
  Constant : Constant  Value=eye(3)
  Constant1 : Constant  Value=eye(3)
  Constant2 : Constant  Value=zeros(3,9)  VectorParams1D=off
  Constant3 : Constant  Value=zeros(3,1)  VectorParams1D=off
  Data Store Read1 : DataStoreRead  DataStoreName=vnav
  Data Store Read3 : DataStoreRead  DataStoreName=P
  Data Store Write : DataStoreWrite  DataStoreName=P
  MATLAB Function1 : MATLAB Function  TreatAsAtomicUnit=on
  MATLAB Function3 : MATLAB Function  TreatAsAtomicUnit=on
  Math Function : Math  Operator=reciprocal  SaturateOnIntegerOverflow=on
  Math Function1 : Math  Operator=square  SaturateOnIntegerOverflow=on
  Matrix Concatenate : Concatenate  Mode=Multidimensional array  ConcatenateDimension=2
  Pad : dspsigops/Pad  padAlong=Rows  dimsToPad=1  valSrc=Specify via dialog  padVal=0  spec=Output size  padNumOutRowsSpecMethod=User-specified  numOutRows=1  padNumOutColsSpecMethod=User-specified  numOutCols=modelDef.numStates  isVarDimsMode=off  padBeginning=0  padEnd=0  outSizeMode=User-specified  outSize=1  padSigAt=End  trunc_flag=None  roundingMode=Floor  overflowMode=off  truncOrWrapMode=Truncate  wrap_flag=None
      settings: SourceProductName=DSP System Toolbox  SourceProductBaseCode=DS
  Product1 : Product  Multiplication=Matrix(*)
  Product2 : Product
  Saturation : Saturate  UpperLimit=100  LowerLimit=0.1
  Scope : Scope
  Scope1 : Scope
  Sum1 : Sum  Inputs=|+-
  update the underlying states : Subsystem
  Out1 : Outport
  wires:
  MATLAB Function1/2(K) -> Product1/1, MATLAB Function3/2(K)
  Pad/1 -> MATLAB Function1/2(H), MATLAB Function3/3(H)
  Math Function1/1 -> Product2/2
  stilltime/1 -> 0.01s to 10s/1
  Saturation/1 -> Scope/1, Math Function1/1
  Math Function/1 -> Saturation/1
  Constant/1 -> Product2/1
  Product1/1 -> update the underlying states/1(" error state estimates")  "errors"
  Product2/1 -> MATLAB Function1/3(R), MATLAB Function3/4(R)
  Data Store Read3/1 -> MATLAB Function1/1(P), MATLAB Function3/1(P)
  Matrix Concatenate/1 -> Pad/1
  MATLAB Function3/1(Pplus) -> Data Store Write/1
  Sum1/1 -> Scope1/1, Product1/2  "nu = dv = vhat - vtrue"
  In1/1 -> Out1/1
  Constant2/1 -> Matrix Concatenate/1
  Constant1/1 -> Matrix Concatenate/2
  0.01s to 10s/1 -> Math Function/1
  Data Store Read1/1 -> Sum1/1
  Constant3/1 -> Sum1/2

== system ImuCalibrator3Pass/thirdPass/readImuData/write SensorTypeIdentifier once ==
  In1 : Inport
  Enable : EnablePort
  Data Store Write : DataStoreWrite  DataStoreName=SensorTypeIdentifier
  wires:
  In1/1 -> Data Store Write/1

== system ImuCalibrator3Pass/firstPass/AINS/compass meas update/update the Cbn with the errors ==
  phi  rotation errors : Inport
  Data Store Read2 : DataStoreRead  DataStoreName=Cbn
  Data Store Write1 : DataStoreWrite  DataStoreName=Cbn
  MATLAB Function : MATLAB Function  TreatAsAtomicUnit=on
  Product2 : Product  Multiplication=Matrix(*)
  Sum : Sum  Inputs=++|
  re-orthonormalization : Subsystem  TreatAsAtomicUnit=on
  wires:
  re-orthonormalization/1(Out1) -> Data Store Write1/1
  Data Store Read2/1 -> Sum/2, Product2/2
  phi  rotation errors/1 -> MATLAB Function/1(inp_vr)
  Sum/1 -> re-orthonormalization/1(In1)
  Product2/1 -> Sum/1
  MATLAB Function/1(res) -> Product2/1  "[phi X]"

== system ImuCalibrator3Pass/firstPass/AINS/gravity meas update/update the Cbn and b_g with the errors ==
  " error state estimates" : Inport
  Data Store Read1 : DataStoreRead  DataStoreName=dw
  Data Store Read2 : DataStoreRead  DataStoreName=Cbn
  Data Store Read3 : DataStoreRead  DataStoreName=rnav
  Data Store Read4 : DataStoreRead  DataStoreName=vnav
  Data Store Read5 : DataStoreRead  DataStoreName=df
  Data Store Read6 : DataStoreRead  DataStoreName=Macc
  Data Store Read7 : DataStoreRead  DataStoreName=Mgyr
  Data Store Write1 : DataStoreWrite  DataStoreName=Cbn
  Data Store Write2 : DataStoreWrite  DataStoreName=dw
  Data Store Write3 : DataStoreWrite  DataStoreName=rnav
  Data Store Write4 : DataStoreWrite  DataStoreName=vnav
  Data Store Write5 : DataStoreWrite  DataStoreName=df
  Data Store Write6 : DataStoreWrite  DataStoreName=Macc
  Data Store Write7 : DataStoreWrite  DataStoreName=Mgyr
  MATLAB Function : MATLAB Function  TreatAsAtomicUnit=on
  Multiport Selector : dspindex/Multiport Selector  rowsOrCols=Rows  idxCellArray={ 1:3, 4:6, 7:9, 10:12, 13:15, 16:24, 25:33 }  idxErrMode=Clip Index
  Product2 : Product  Multiplication=Matrix(*)
  Reshape : Reshape  OutputDimensionality=Customize  OutputDimensions=[3,3]
  Reshape1 : Reshape  OutputDimensionality=Customize  OutputDimensions=[3,3]
  Sum{,1..6} (7 alike) : Sum  Inputs=++|
  re-orthonormalization : Subsystem  TreatAsAtomicUnit=on
  wires:
  MATLAB Function/1(res) -> Product2/1  "[phi X]"
  Product2/1 -> Sum/1
  Sum/1 -> re-orthonormalization/1(In1)
  Data Store Read2/1 -> Product2/2, Sum/2
  re-orthonormalization/1(Out1) -> Data Store Write1/1
  Multiport Selector/1 -> MATLAB Function/1(inp_vr)  "phi rotation errors"
  Data Store Read1/1 -> Sum1/2
  Sum1/1 -> Data Store Write2/1
  Multiport Selector/2 -> Sum1/1  "gyro bias errors"
  " error state estimates"/1 -> Multiport Selector/1
  Sum2/1 -> Data Store Write3/1
  Data Store Read3/1 -> Sum2/2
  Data Store Read4/1 -> Sum3/2
  Sum3/1 -> Data Store Write4/1
  Multiport Selector/3 -> Sum2/1
  Multiport Selector/4 -> Sum3/1
  Sum4/1 -> Data Store Write5/1
  Data Store Read5/1 -> Sum4/2
  Multiport Selector/5 -> Sum4/1
  Data Store Read6/1 -> Sum5/2
  Sum5/1 -> Data Store Write6/1
  Sum6/1 -> Data Store Write7/1
  Data Store Read7/1 -> Sum6/2
  Multiport Selector/6 -> Reshape/1
  Reshape/1 -> Sum5/1
  Multiport Selector/7 -> Reshape1/1
  Reshape1/1 -> Sum6/1

== system ImuCalibrator3Pass/firstPass/AINS/initialize states and covariances/INITIALIZED = 1 ==
  Enable : EnablePort  ShowOutputPort=on
  Constant : Constant
  Data Store Write : DataStoreWrite  DataStoreName=INITIALIZED
  Out1 : Outport  OutputWhenDisabled=reset  InitialOutput=false
  wires:
  Constant/1 -> Data Store Write/1
  Enable/1 -> Out1/1

== system ImuCalibrator3Pass/firstPass/AINS/initialize states and covariances/calc Cbn ==
  f^b : Inport
  Enable : EnablePort  ShowOutputPort=on
  Constant : Constant  Value=[1 0 0]
  Cross Product : vrlib/Utilities/Cross Product
      settings: SourceProductBaseCode=VR
  Cross Product1 : vrlib/Utilities/Cross Product
      settings: SourceProductBaseCode=VR
  Gain : Gain  Gain=-1
  Matrix Concatenate : Concatenate  NumInputs=3  Mode=Multidimensional array
  Normalize Vector : vrlib/Utilities/Normalize Vector  maxzero=0
      settings: SourceProductName=Simulink 3D Animation  SourceProductBaseCode=VR
  Normalize Vector1 : vrlib/Utilities/Normalize Vector  maxzero=0
      settings: SourceProductName=Simulink 3D Animation  SourceProductBaseCode=VR
  Normalize Vector2 : vrlib/Utilities/Normalize Vector  maxzero=0
      settings: SourceProductName=Simulink 3D Animation  SourceProductBaseCode=VR
  Out1 : Outport  OutputWhenDisabled=reset  InitialOutput=false
  Cbn : Outport  Port=2
  wires:
  f^b/1 -> Gain/1  "up"
  Gain/1 -> Normalize Vector2/1, Cross Product1/2, Cross Product/1  "down^b"
  Constant/1 -> Cross Product/2
  Cross Product/1 -> Normalize Vector1/1, Cross Product1/1  "east^b"
  Cross Product1/1 -> Normalize Vector/1  "north^b"
  Normalize Vector/1 -> Matrix Concatenate/1
  Normalize Vector1/1 -> Matrix Concatenate/2
  Normalize Vector2/1 -> Matrix Concatenate/3
  Matrix Concatenate/1 -> Cbn/1
  Enable/1 -> Out1/1

== system ImuCalibrator3Pass/firstPass/AINS/initialize states and covariances/set P ==
  Enable : EnablePort  ShowOutputPort=on
  Data Store Write : DataStoreWrite  DataStoreName=P
  Gain : Gain
  Gain2 : Gain
  Gain3 : Gain
  MATLAB Function1 : MATLAB Function  TreatAsAtomicUnit=on
  "initial position error, m rms" : Constant  Value=[0.01; 0.01; 0.01]  VectorParams1D=off
  "initial rotation error, rad rms" : Constant  Value=[0.1; 0.1; 0.1]  VectorParams1D=off
  "initial vel error, m/s" : Constant  Value=[0.01; 0.01; 0.01]  VectorParams1D=off
  Out1 : Outport  OutputWhenDisabled=reset  InitialOutput=false
  wires:
  MATLAB Function1/1(P0) -> Data Store Write/1
  "initial rotation error, rad rms"/1 -> Gain/1
  "initial position error, m rms"/1 -> Gain2/1
  Gain/1 -> MATLAB Function1/1(initialRotUncert)
  Gain2/1 -> MATLAB Function1/2(initialPosUncert)
  "initial vel error, m/s"/1 -> Gain3/1
  Gain3/1 -> MATLAB Function1/3(initialVelUncert)
  Enable/1 -> Out1/1

== system ImuCalibrator3Pass/firstPass/AINS/initialize states and covariances/set states ==
  Cbn : Inport
  Enable : EnablePort  ShowOutputPort=on
  Constant{,1..3} (4 alike) : Constant  Value=[0;0;0]
  Constant4 : Constant  Value=[0 0 0; 0 0 0; 0 0 0]  VectorParams1D=off
  Constant5 : Constant  Value=[0 0 0; 0 0 0; 0 0 0]  VectorParams1D=off
  Constant6 : Constant  Value=[1 0 0; 0 1 0; 0 0 1]  VectorParams1D=off
  Constant7 : Constant  Value=[1 0 0; 0 1 0; 0 0 1]  VectorParams1D=off
  Constant8 : Constant  Value=[0 0 0; 0 0 0; 0 0 0]  VectorParams1D=off
  Data Store Write : DataStoreWrite  DataStoreName=dw
  Data Store Write1 : DataStoreWrite  DataStoreName=df
  Data Store Write2 : DataStoreWrite  DataStoreName=vnav
  Data Store Write3 : DataStoreWrite  DataStoreName=rnav
  Data Store Write4 : DataStoreWrite  DataStoreName=Macc
  Data Store Write5 : DataStoreWrite  DataStoreName=Mgyr
  Data Store Write6 : DataStoreWrite  DataStoreName=IplusMinv_acc
  Data Store Write7 : DataStoreWrite  DataStoreName=IplusMinv_gyr
  Data Store Write8 : DataStoreWrite  DataStoreName=Cbn
  Data Store Write9 : DataStoreWrite  DataStoreName=Ggyr
  Out1 : Outport  OutputWhenDisabled=reset  InitialOutput=false
  wires:
  Constant/1 -> Data Store Write/1
  Constant1/1 -> Data Store Write1/1
  Constant2/1 -> Data Store Write2/1
  Constant3/1 -> Data Store Write3/1
  Constant4/1 -> Data Store Write4/1
  Constant5/1 -> Data Store Write5/1
  Constant6/1 -> Data Store Write6/1
  Constant7/1 -> Data Store Write7/1
  Enable/1 -> Out1/1
  Cbn/1 -> Data Store Write8/1
  Constant8/1 -> Data Store Write9/1
